simulink model "wind_turbine_with_wind"  (Simulink 7.7)
settings: Solver=ode45  StartTime=0.0  StopTime=inf  RelTol=1e-3
values from neighbouring files (symbols this model uses):
  q = [x2;y2;c2;x3;y3;z3;a3;b3;c3;x4;y4;z4;b4;c4;x5;y5;z5;b5;c5;a6;b6;c6;a7;xSun;ySun;zSun;bSun;cSun;xPla1;yPla1;zPla1;bPla1;cPla1;xPla2;yPla2;zPla2;bPla2;cPla2;xPla3;yPla3;zPla3;bPla3;cPla3;xSecSt;ySecSt;zSecSt;bSecSt;cSecSt;a4;a5;aSun;aPla1;aPla2;aPla3;aSecSt;]    [environment.m]
undefined symbols (not defined in the file or in its folder): B, DU21, DU25, DU30, DU35, DU40, NACA64, rho
settings Model: Creator=imac  LastModifiedBy=aitor

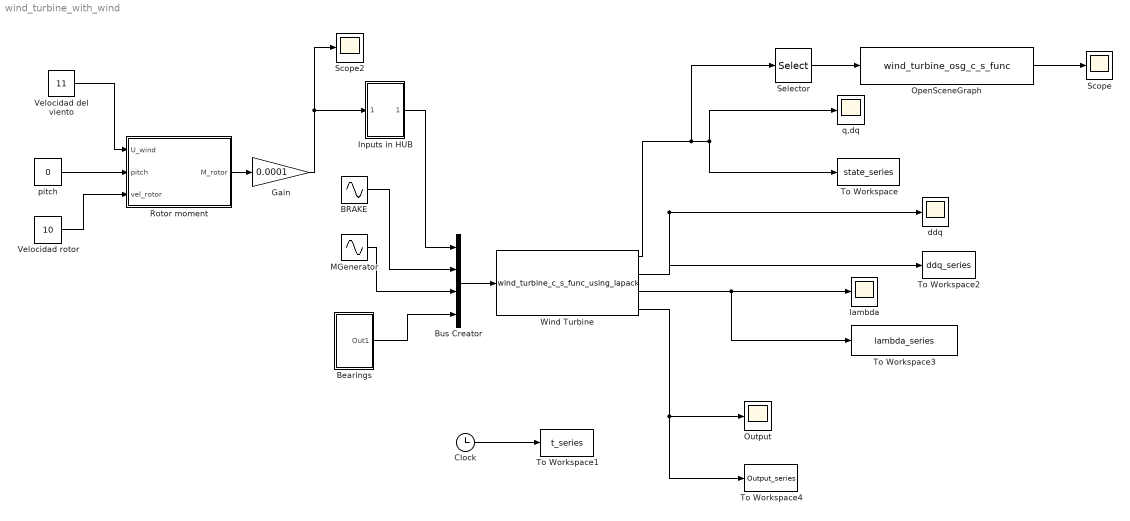
== system wind_turbine_with_wind ==
  BRAKE : Sin  Amplitude=0  Frequency=0  Phase=pi/2  SampleTime=0
  Bearings : Subsystem
  Bus Creator : BusCreator
  Clock : Clock
  Gain : Gain  Gain=0.0001
  Inputs in HUB : Subsystem
  MGenerator : Sin  Amplitude=0  Frequency=0  Phase=pi/2  SampleTime=0
  OpenSceneGraph : S-Function  FunctionName=wind_turbine_osg_c_s_func  EnableBusSupport=off
  Output : Scope
      settings: YMin=0  YMax=1300  SaveName=ScopeData3  SampleInput=on  SampleTime=0.01
  Rotor moment : Stateflow chart  LoadFcn=|  TreatAsAtomicUnit=on
      | load ./profiles/DU21.dat;  
      | load ./profiles/DU25.dat;  
      | load ./profiles/DU30.dat;  
      | load ./profiles/DU35.dat;  
      | load ./profiles/DU40.dat;  
      | load ./profiles/NACA64.dat;
      | B=3;                       
      | rho=1.225 ;
  Scope : Scope
      settings: SaveName=ScopeData4
  Scope2 : Scope
      settings: YMin=524.269  YMax=524.269  SaveName=ScopeData6
  Selector : Selector  InputPortWidth=2*length(q)  IndexOptions=Index vector (dialog)  Indices=1:1:length(q)  OutputSizes=1
  To Workspace : ToWorkspace  VariableName=state_series  SampleTime=0.01  SaveFormat=Array
  To Workspace1 : ToWorkspace  VariableName=t_series  SampleTime=0.01  SaveFormat=Array
  To Workspace2 : ToWorkspace  VariableName=ddq_series  SampleTime=0.01  SaveFormat=Array
  To Workspace3 : ToWorkspace  VariableName=lambda_series  SampleTime=0.01  SaveFormat=Array
  To Workspace4 : ToWorkspace  VariableName=Output_series  SampleTime=0.01  SaveFormat=Array
  Velocidad del viento : Constant  Value=11
  Velocidad rotor : Constant  Value=10
  Wind Turbine : S-Function  FunctionName=wind_turbine_c_s_func_using_lapack  Parameters=q dq param  EnableBusSupport=off
      mask Type: S-function: mycsfunc
      mask Description: This is a S-function that does the continuous state space system.
      mask Display: disp('[M , Phi_q''] [ddq]\n[Phi_q , 0] [lambda]\n=\n [Q ] \n   [gamma] ');
  ddq : Scope
      settings: YMin=-500  YMax=300  SampleInput=on  SampleTime=0.01
  lambda : Scope
      settings: YMin=-1750  YMax=1000  SaveName=ScopeData2  SampleInput=on  SampleTime=0.01
  pitch : Constant  Value=0
  q,dq : Scope
      settings: YMin=-0.035  YMax=0.045  SampleInput=on  SampleTime=0.01
  wires:
  Clock/1 -> To Workspace1/1
  Wind Turbine/1 -> q,dq/1, To Workspace/1, Selector/1
  Wind Turbine/2 -> ddq/1, To Workspace2/1
  Wind Turbine/3 -> lambda/1, To Workspace3/1
  Wind Turbine/4 -> Output/1, To Workspace4/1
  Selector/1 -> OpenSceneGraph/1
  OpenSceneGraph/1 -> Scope/1
  Inputs in HUB/1(Out1) -> Bus Creator/1
  Bus Creator/1 -> Wind Turbine/1
  BRAKE/1 -> Bus Creator/2
  MGenerator/1 -> Bus Creator/3
  Bearings/1(Out1) -> Bus Creator/4
  Velocidad del viento/1 -> Rotor moment/1(U_wind)
  pitch/1 -> Rotor moment/2(pitch)
  Velocidad rotor/1 -> Rotor moment/3(vel_rotor)
  Rotor moment/1(M_rotor) -> Gain/1
  Gain/1 -> Scope2/1, Inputs in HUB/1(In1)

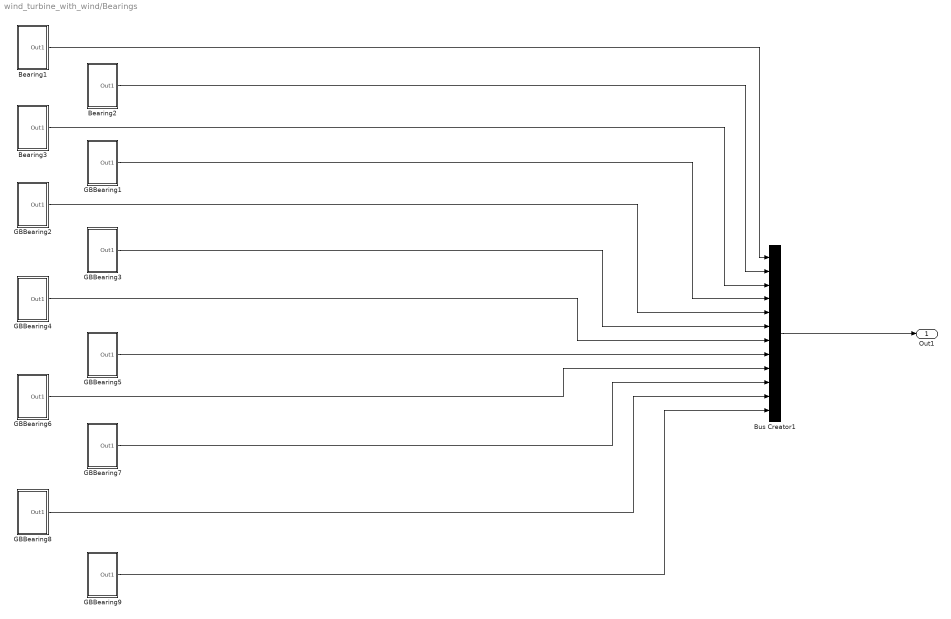
== system wind_turbine_with_wind/Bearings ==
  " GBBearing2" : Subsystem
  Bearing1 : Subsystem
  Bearing2 : Subsystem
  Bearing3 : Subsystem
  Bus Creator1 : BusCreator  Inputs=12
  GBBearing1 : Subsystem
  GBBearing3 : Subsystem
  GBBearing4 : Subsystem
  GBBearing5 : Subsystem
  GBBearing6 : Subsystem
  GBBearing7 : Subsystem
  GBBearing8 : Subsystem
  GBBearing9 : Subsystem
  Out1 : Outport
  wires:
  Bearing1/1(Out1) -> Bus Creator1/1
  Bearing2/1(Out1) -> Bus Creator1/2
  Bearing3/1(Out1) -> Bus Creator1/3
  GBBearing1/1(Out1) -> Bus Creator1/4
  Bus Creator1/1 -> Out1/1
  " GBBearing2"/1(Out1) -> Bus Creator1/5
  GBBearing3/1(Out1) -> Bus Creator1/6
  GBBearing4/1(Out1) -> Bus Creator1/7
  GBBearing5/1(Out1) -> Bus Creator1/8
  GBBearing6/1(Out1) -> Bus Creator1/9
  GBBearing7/1(Out1) -> Bus Creator1/10
  GBBearing8/1(Out1) -> Bus Creator1/11
  GBBearing9/1(Out1) -> Bus Creator1/12

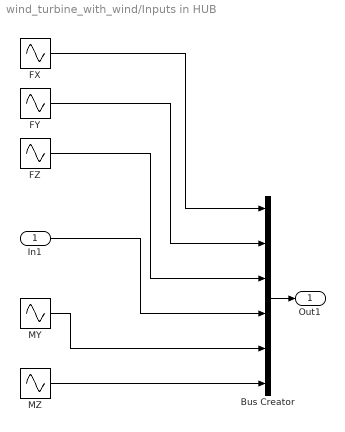
== system wind_turbine_with_wind/Inputs in HUB ==
  In1 : Inport
  Bus Creator : BusCreator  Inputs=6
  FX : Sin  Description=FX  Amplitude=0  Frequency=0  Phase=pi/2  SampleTime=0
  FY : Sin  Amplitude=0  Frequency=0  Phase=pi/2  SampleTime=0
  FZ : Sin  Amplitude=0  Frequency=0  Phase=pi/2  SampleTime=0
  MY : Sin  Amplitude=0  Frequency=0  Phase=pi/2  SampleTime=0
  MZ : Sin  Amplitude=0  Frequency=0  Phase=pi/2  SampleTime=0
  Out1 : Outport
  wires:
  FX/1 -> Bus Creator/1
  FY/1 -> Bus Creator/2
  MY/1 -> Bus Creator/5
  MZ/1 -> Bus Creator/6
  FZ/1 -> Bus Creator/3
  Bus Creator/1 -> Out1/1
  In1/1 -> Bus Creator/4

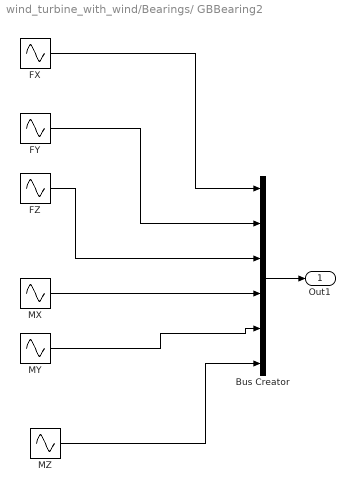
== system wind_turbine_with_wind/Bearings/ GBBearing2 ==
  Bus Creator : BusCreator  Inputs=6
  FX : Sin  Description=FX  Amplitude=0  Frequency=0  Phase=pi/2  SampleTime=0
  FY : Sin  Amplitude=0  Frequency=0  Phase=pi/2  SampleTime=0
  FZ : Sin  Amplitude=0  Frequency=0  Phase=pi/2  SampleTime=0
  MX : Sin  Amplitude=0  Frequency=0  Phase=pi/2  SampleTime=0
  MY : Sin  Amplitude=0  Frequency=0  Phase=pi/2  SampleTime=0
  MZ : Sin  Amplitude=0  Frequency=0  Phase=pi/2  SampleTime=0
  Out1 : Outport
  wires:
  FX/1 -> Bus Creator/1
  FY/1 -> Bus Creator/2
  MX/1 -> Bus Creator/4
  MY/1 -> Bus Creator/5
  MZ/1 -> Bus Creator/6
  FZ/1 -> Bus Creator/3
  Bus Creator/1 -> Out1/1

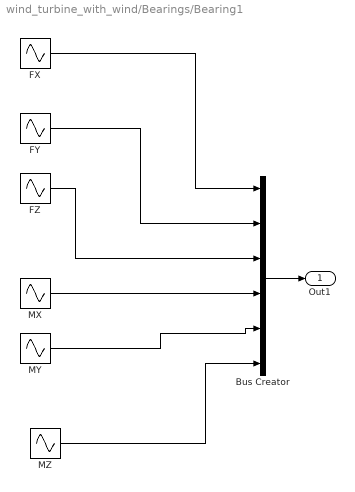
== system wind_turbine_with_wind/Bearings/Bearing1 ==
  Bus Creator : BusCreator  Inputs=6
  FX : Sin  Description=FX  Amplitude=0  Frequency=0  Phase=pi/2  SampleTime=0
  FY : Sin  Amplitude=0  Frequency=0  Phase=pi/2  SampleTime=0
  FZ : Sin  Amplitude=0  Frequency=0  Phase=pi/2  SampleTime=0
  MX : Sin  Amplitude=0  Frequency=0  Phase=pi/2  SampleTime=0
  MY : Sin  Amplitude=0  Frequency=0  Phase=pi/2  SampleTime=0
  MZ : Sin  Amplitude=0  Frequency=0  Phase=pi/2  SampleTime=0
  Out1 : Outport
  wires:
  FX/1 -> Bus Creator/1
  FY/1 -> Bus Creator/2
  MX/1 -> Bus Creator/4
  MY/1 -> Bus Creator/5
  MZ/1 -> Bus Creator/6
  FZ/1 -> Bus Creator/3
  Bus Creator/1 -> Out1/1

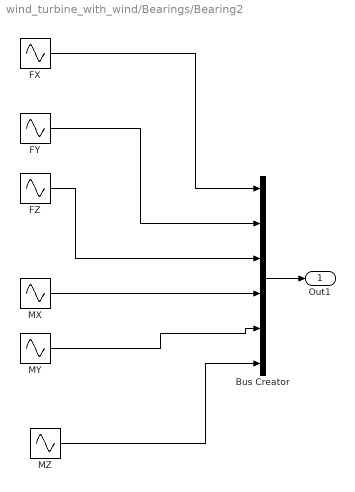
== system wind_turbine_with_wind/Bearings/Bearing2 ==
  Bus Creator : BusCreator  Inputs=6
  FX : Sin  Description=FX  Amplitude=0  Frequency=0  Phase=pi/2  SampleTime=0
  FY : Sin  Amplitude=0  Frequency=0  Phase=pi/2  SampleTime=0
  FZ : Sin  Amplitude=0  Frequency=pi/2  SampleTime=0
  MX : Sin  Amplitude=0  Frequency=0  Phase=pi/2  SampleTime=0
  MY : Sin  Amplitude=0  Frequency=0  Phase=pi/2  SampleTime=0
  MZ : Sin  Amplitude=0  Frequency=0  Phase=pi/2  SampleTime=0
  Out1 : Outport
  wires:
  FX/1 -> Bus Creator/1
  FY/1 -> Bus Creator/2
  MX/1 -> Bus Creator/4
  MY/1 -> Bus Creator/5
  MZ/1 -> Bus Creator/6
  FZ/1 -> Bus Creator/3
  Bus Creator/1 -> Out1/1

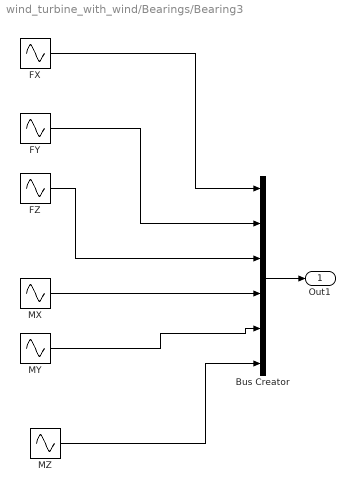
== system wind_turbine_with_wind/Bearings/Bearing3 ==
  Bus Creator : BusCreator  Inputs=6
  FX : Sin  Description=FX  Amplitude=0  Frequency=0  Phase=pi/2  SampleTime=0
  FY : Sin  Amplitude=0  Frequency=0  Phase=pi/2  SampleTime=0
  FZ : Sin  Amplitude=0  Frequency=0  Phase=pi/2  SampleTime=0
  MX : Sin  Amplitude=0  Frequency=0  Phase=pi/2  SampleTime=0
  MY : Sin  Amplitude=0  Frequency=0  Phase=pi/2  SampleTime=0
  MZ : Sin  Amplitude=0  Frequency=0  Phase=pi/2  SampleTime=0
  Out1 : Outport
  wires:
  FX/1 -> Bus Creator/1
  FY/1 -> Bus Creator/2
  MX/1 -> Bus Creator/4
  MY/1 -> Bus Creator/5
  MZ/1 -> Bus Creator/6
  FZ/1 -> Bus Creator/3
  Bus Creator/1 -> Out1/1

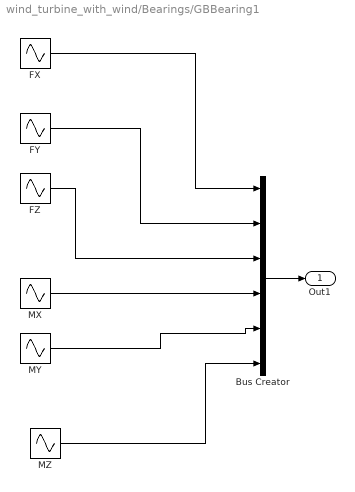
== system wind_turbine_with_wind/Bearings/GBBearing1 ==
  Bus Creator : BusCreator  Inputs=6
  FX : Sin  Description=FX  Amplitude=0  Frequency=0  Phase=pi/2  SampleTime=0
  FY : Sin  Amplitude=0  Frequency=0  Phase=pi/2  SampleTime=0
  FZ : Sin  Amplitude=0  Frequency=pi/2  SampleTime=0
  MX : Sin  Amplitude=0  Frequency=0  Phase=pi/2  SampleTime=0
  MY : Sin  Amplitude=0  Frequency=0  Phase=pi/2  SampleTime=0
  MZ : Sin  Amplitude=0  Frequency=0  Phase=pi/2  SampleTime=0
  Out1 : Outport
  wires:
  FX/1 -> Bus Creator/1
  FY/1 -> Bus Creator/2
  MX/1 -> Bus Creator/4
  MY/1 -> Bus Creator/5
  MZ/1 -> Bus Creator/6
  FZ/1 -> Bus Creator/3
  Bus Creator/1 -> Out1/1

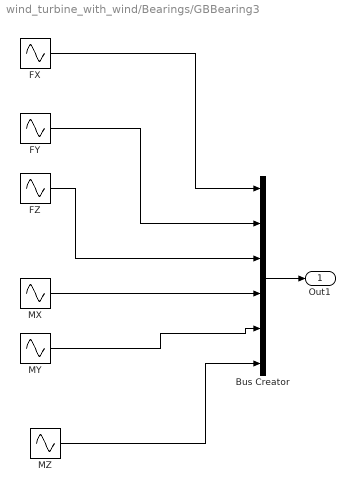
== system wind_turbine_with_wind/Bearings/GBBearing3 ==
  Bus Creator : BusCreator  Inputs=6
  FX : Sin  Description=FX  Amplitude=0  Frequency=0  Phase=pi/2  SampleTime=0
  FY : Sin  Amplitude=0  Frequency=0  Phase=pi/2  SampleTime=0
  FZ : Sin  Amplitude=0  Frequency=0  Phase=pi/2  SampleTime=0
  MX : Sin  Amplitude=0  Frequency=0  Phase=pi/2  SampleTime=0
  MY : Sin  Amplitude=0  Frequency=0  Phase=pi/2  SampleTime=0
  MZ : Sin  Amplitude=0  Frequency=0  Phase=pi/2  SampleTime=0
  Out1 : Outport
  wires:
  FX/1 -> Bus Creator/1
  FY/1 -> Bus Creator/2
  MX/1 -> Bus Creator/4
  MY/1 -> Bus Creator/5
  MZ/1 -> Bus Creator/6
  FZ/1 -> Bus Creator/3
  Bus Creator/1 -> Out1/1

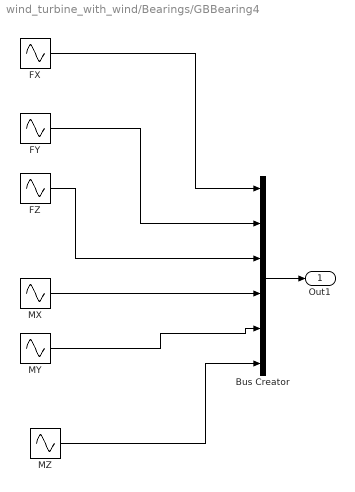
== system wind_turbine_with_wind/Bearings/GBBearing4 ==
  Bus Creator : BusCreator  Inputs=6
  FX : Sin  Description=FX  Amplitude=0  Frequency=0  Phase=pi/2  SampleTime=0
  FY : Sin  Amplitude=0  Frequency=0  Phase=pi/2  SampleTime=0
  FZ : Sin  Amplitude=0  Frequency=0  Phase=pi/2  SampleTime=0
  MX : Sin  Amplitude=0  Frequency=0  Phase=pi/2  SampleTime=0
  MY : Sin  Amplitude=0  Frequency=0  Phase=pi/2  SampleTime=0
  MZ : Sin  Amplitude=0  Frequency=0  Phase=pi/2  SampleTime=0
  Out1 : Outport
  wires:
  FX/1 -> Bus Creator/1
  FY/1 -> Bus Creator/2
  MX/1 -> Bus Creator/4
  MY/1 -> Bus Creator/5
  MZ/1 -> Bus Creator/6
  FZ/1 -> Bus Creator/3
  Bus Creator/1 -> Out1/1

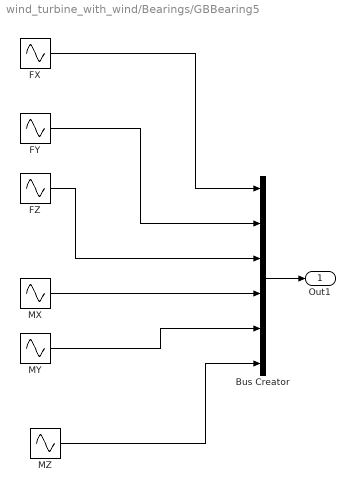
== system wind_turbine_with_wind/Bearings/GBBearing5 ==
  Bus Creator : BusCreator  Inputs=6
  FX : Sin  Description=FX  Amplitude=0  Frequency=0  Phase=pi/2  SampleTime=0
  FY : Sin  Amplitude=0  Frequency=0  Phase=pi/2  SampleTime=0
  FZ : Sin  Amplitude=0  Frequency=0  Phase=pi/2  SampleTime=0
  MX : Sin  Amplitude=0  Frequency=0  Phase=pi/2  SampleTime=0
  MY : Sin  Amplitude=0  Frequency=0  Phase=pi/2  SampleTime=0
  MZ : Sin  Amplitude=0  Frequency=0  Phase=pi/2  SampleTime=0
  Out1 : Outport
  wires:
  FX/1 -> Bus Creator/1
  FY/1 -> Bus Creator/2
  MX/1 -> Bus Creator/4
  MY/1 -> Bus Creator/5
  MZ/1 -> Bus Creator/6
  FZ/1 -> Bus Creator/3
  Bus Creator/1 -> Out1/1

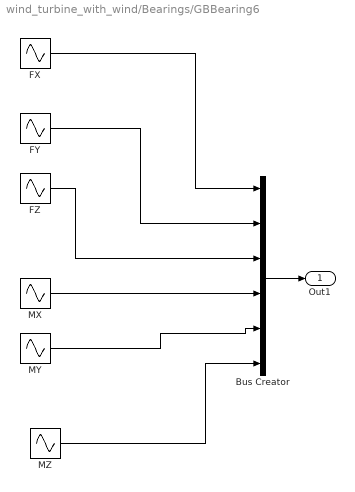
== system wind_turbine_with_wind/Bearings/GBBearing6 ==
  Bus Creator : BusCreator  Inputs=6
  FX : Sin  Description=FX  Amplitude=0  Frequency=0  Phase=pi/2  SampleTime=0
  FY : Sin  Amplitude=0  Frequency=0  Phase=pi/2  SampleTime=0
  FZ : Sin  Amplitude=0  Frequency=0  Phase=pi/2  SampleTime=0
  MX : Sin  Amplitude=0  Frequency=0  Phase=pi/2  SampleTime=0
  MY : Sin  Amplitude=0  Frequency=0  Phase=pi/2  SampleTime=0
  MZ : Sin  Amplitude=0  Frequency=0  Phase=pi/2  SampleTime=0
  Out1 : Outport
  wires:
  FX/1 -> Bus Creator/1
  FY/1 -> Bus Creator/2
  MX/1 -> Bus Creator/4
  MY/1 -> Bus Creator/5
  MZ/1 -> Bus Creator/6
  FZ/1 -> Bus Creator/3
  Bus Creator/1 -> Out1/1

== system wind_turbine_with_wind/Bearings/GBBearing7 ==
  Bus Creator : BusCreator  Inputs=6
  FX : Sin  Description=FX  Amplitude=0  Frequency=0  Phase=pi/2  SampleTime=0
  FY : Sin  Amplitude=0  Frequency=0  Phase=pi/2  SampleTime=0
  FZ : Sin  Amplitude=0  Frequency=100  Phase=pi/2  SampleTime=0
  MX : Sin  Amplitude=0  Frequency=0  Phase=pi/2  SampleTime=0
  MY : Sin  Amplitude=0  Frequency=0  Phase=pi/2  SampleTime=0
  MZ : Sin  Amplitude=0  Frequency=0  Phase=pi/2  SampleTime=0
  Out1 : Outport
  wires:
  FX/1 -> Bus Creator/1
  FY/1 -> Bus Creator/2
  MX/1 -> Bus Creator/4
  MY/1 -> Bus Creator/5
  MZ/1 -> Bus Creator/6
  FZ/1 -> Bus Creator/3
  Bus Creator/1 -> Out1/1

== system wind_turbine_with_wind/Bearings/GBBearing8 ==
  Bus Creator : BusCreator  Inputs=6
  FX : Sin  Description=FX  Amplitude=0  Frequency=0  Phase=pi/2  SampleTime=0
  FY : Sin  Amplitude=0  Frequency=0  Phase=pi/2  SampleTime=0
  FZ : Sin  Amplitude=0  Frequency=100  Phase=pi/2  SampleTime=0
  MX : Sin  Amplitude=0  Frequency=0  Phase=pi/2  SampleTime=0
  MY : Sin  Amplitude=0  Frequency=0  Phase=pi/2  SampleTime=0
  MZ : Sin  Amplitude=0  Frequency=0  Phase=pi/2  SampleTime=0
  Out1 : Outport
  wires:
  FX/1 -> Bus Creator/1
  FY/1 -> Bus Creator/2
  MX/1 -> Bus Creator/4
  MY/1 -> Bus Creator/5
  MZ/1 -> Bus Creator/6
  FZ/1 -> Bus Creator/3
  Bus Creator/1 -> Out1/1

== system wind_turbine_with_wind/Bearings/GBBearing9 ==
  Bus Creator : BusCreator  Inputs=6
  FX : Sin  Description=FX  Amplitude=0  Frequency=0  Phase=pi/2  SampleTime=0
  FY : Sin  Amplitude=0  Frequency=0  Phase=pi/2  SampleTime=0
  FZ : Sin  Amplitude=0  Frequency=0  Phase=pi/2  SampleTime=0
  MX : Sin  Amplitude=0  Frequency=0  Phase=pi/2  SampleTime=0
  MY : Sin  Amplitude=0  Frequency=0  Phase=pi/2  SampleTime=0
  MZ : Sin  Amplitude=0  Frequency=0  Phase=pi/2  SampleTime=0
  Out1 : Outport
  wires:
  FX/1 -> Bus Creator/1
  FY/1 -> Bus Creator/2
  MX/1 -> Bus Creator/4
  MY/1 -> Bus Creator/5
  MZ/1 -> Bus Creator/6
  FZ/1 -> Bus Creator/3
  Bus Creator/1 -> Out1/1

== matlab function Rotor moment ==
  data: U_wind input double; pitch input double; vel_rotor input double; M_rotor output double; DU21 parameter double; DU25 parameter double; DU30 parameter double; DU35 parameter double; DU40 parameter double; NACA64 parameter double; B parameter double; rho parameter double
function M_rotor  = BEM_pala (U_wind,pitch,vel_rotor,DU21,DU25,DU30,DU35,DU40,NACA64,B,rho)
coder.extrinsic('BEM');
U=U_wind;
vel=vel_rotor;
omega=vel*2*pi/60;

r=[8.33 11.75 15.85 19.95 24.05 28.15 32.25 36.35 40.45 44.55 48.65 52.75 56.17 58.90 61.63];
c=[4.17 4.56 4.65 4.46 4.25 4.01 3.75 3.50 3.26 3.01 2.76 2.52 2.31 2.09 1.42];
thetar=[13.31 13.31 11.48 10.16 9.01 7.80 6.54 5.36 4.19 3.13 2.32 1.53 0.86 0.37 0.11];
thetap0=pitch;
tipo_perfil=[5 5 4 4 3 2 2 1 1 6 6 6 6 6 6];
%tipos de perfiles 1=DU21 2=DU25 3=DU30 4=DU35 5=DU40 6=NACA64];
dr=[2.73 4.10 4.10 4.10 4.10 4.10 4.10 4.10 4.10 4.10 4.10 4.10 2.73 2.73 2.73];

resultados=zeros(length(tipo_perfil));
perfil=[];
for i=1:1:15,
	switch tipo_perfil(i),
	case 1,
		perfil=DU21;
	case 2,
		perfil=DU25;
	case 3
		perfil=DU30;
	case 4,
		perfil=DU35;
	case 5
		perfil=DU40;
	case 6 
		perfil=NACA64;
    end
   
dQ=BEM(U,omega,r(1,i),dr(1,i),c(1,i),thetap0,thetar(1,i),perfil,B,rho);
resultados(i)=dQ;
end
M_rotor=sum(resultados(:,1));
